simulink model "test_model"  (R2023a)
settings: Solver=ode5  StartTime=0.0  StopTime=10  FixedStep=0.002  RelTol=1e-3
undefined symbols (not defined in the file or in its folder): f
libraries: sldrtlib x3, instrumentlib x1
settings Model: Creator=DELL  LastModifiedBy=DELL
settings HardwareCC: ProdBitPerLong=64  ProdHWDeviceType=Intel->x86-64 (Linux 64)
settings ModelReferenceCC: EnableRefExpFcnMdlSchedulingChecks=on
settings RTWCC: Description=Simulink Desktop Real-Time  SystemTargetFile=sldrt.tlc  TemplateMakefile=sldrt.tmf  RTWCompilerOptimization=on
settings CodeAppCC: MaxIdLength=95
settings SimulinkDesktopRealTimeCC: TargetLibSuffix=_sldrt.a  TargetPreCompLibLocation=C:\Program Files\MATLAB\R2023a\toolbox\sldrt\lib\win64

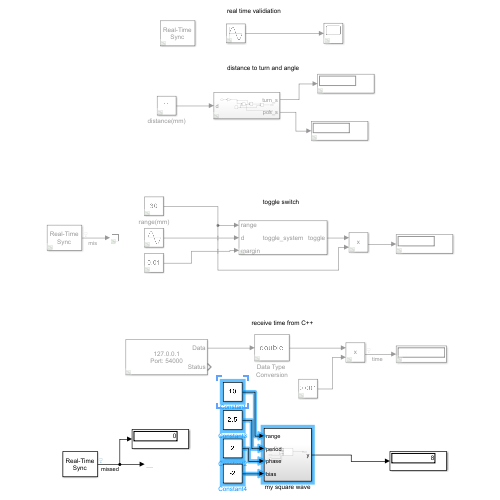
[thumbnail: Simulink's stored preview of the top-level diagram]
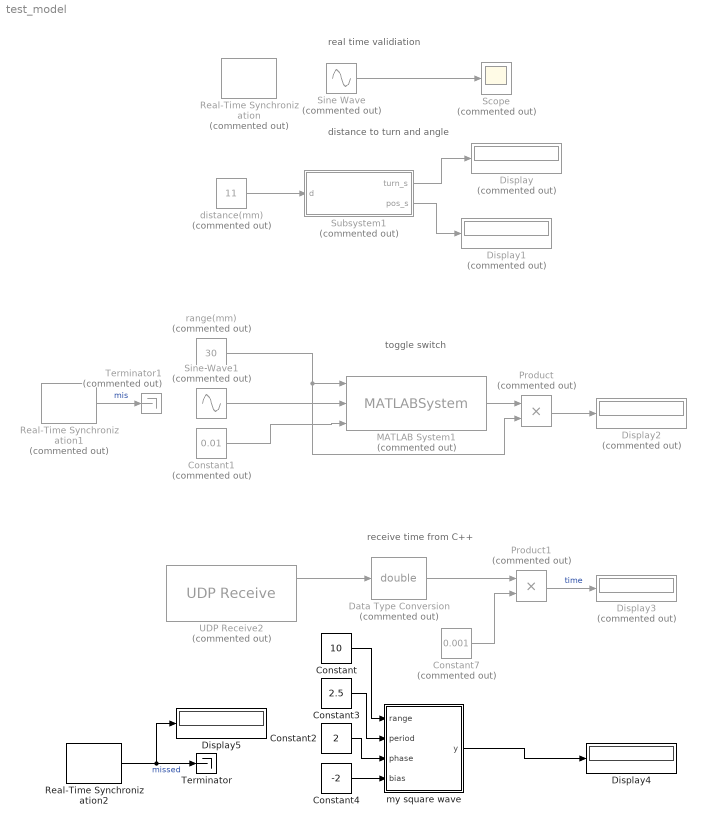
== system test_model ==
  note: real time validiation
  note: toggle switch
  note: distance to turn and angle
  note: receive time from C++
  Constant : Constant  Value=10
  Constant1 : Constant  Commented=on  Value=0.01
  Constant2 : Constant  Value=2
  Constant3 : Constant  Value=2.5
  Constant4 : Constant  Value=-2
  Constant7 : Constant  Commented=on  Value=0.001
  Data Type Conversion : DataTypeConversion  Commented=on  OutDataTypeStr=double  SaturateOnIntegerOverflow=off  RndMeth=Floor
  Display{,1..3} (4 alike) : Display  Commented=on
  Display4 : Display
  Display5 : Display
  MATLAB System1 : MATLABSystem  Commented=on  System=toggle_system  SimulateUsing=Code generation
      mask Type: toggle_system
      mask Display:
      | disp('toggle_system');
      | port_label('input',1,'range');
      | port_label('input',2,'d');
      | port_label('input',3,'margin');
      | port_label('output',1,'toggle');
  Product : Product  Commented=on
  Product1 : Product  Commented=on
  Real-Time Synchronization : sldrtlib/Real-Time Synchronization  Commented=on  SampleTime=0.01  MaxMissedTicks=10  ShowMissedTicks=off  YieldWhenWaiting=off
  Real-Time Synchronization1 : sldrtlib/Real-Time Synchronization  Commented=on  SampleTime=0.1  MaxMissedTicks=10  ShowMissedTicks=on  YieldWhenWaiting=off
  Real-Time Synchronization2 : sldrtlib/Real-Time Synchronization  SampleTime=0.002  MaxMissedTicks=inf  ShowMissedTicks=on  YieldWhenWaiting=off
  Scope : Scope  Commented=on
  Sine Wave : Sin  Commented=on
  Sine Wave1 : Sin  Commented=on  Amplitude=30  SampleTime=0
  Subsystem1 : Subsystem  Commented=on
  Terminator : Terminator
  Terminator1 : Terminator  Commented=on
  UDP Receive2 : instrumentlib/UDP Receive  Commented=on  LocalAddress=127.0.0.1  LocalPort=54000  EnablePortSharing=off  Host=127.0.0.1  Port=8080  GetLatestData=on  DataSize=1  DataType=uint32  ASCIIFormatting=%f,  Terminator=LF  CustomTerminator=10  ByteOrder=little-endian  EnableBlockingMode=off  Timeout=1  SampleTime=0.01  SimulateUsing=Interpreted execution
  distance(mm) : Constant  Commented=on  Value=11
  my square wave : Subsystem
  range(mm) : Constant  Commented=on  Value=30
  wires:
  Sine Wave/1 -> Scope/1
  distance(mm)/1 -> Subsystem1/1(d)
  Subsystem1/1(turn_s) -> Display/1
  Subsystem1/2(pos_s) -> Display1/1
  MATLAB System1/1 -> Product/1
  Sine Wave1/1 -> MATLAB System1/2
  Product1/1 -> Display3/1  "time"
  Data Type Conversion/1 -> Product1/1
  Constant7/1 -> Product1/2
  UDP Receive2/1 -> Data Type Conversion/1
  Product/1 -> Display2/1
  Constant1/1 -> MATLAB System1/3
  range(mm)/1 -> Product/2, MATLAB System1/1
  Real-Time Synchronization2/1 -> Display5/1, Terminator/1  "missed"
  Real-Time Synchronization1/1 -> Terminator1/1  "mis"
  Constant/1 -> my square wave/1(range)
  Constant3/1 -> my square wave/2(period)
  Constant2/1 -> my square wave/3(phase)
  my square wave/1(y) -> Display4/1
  Constant4/1 -> my square wave/4(bias)

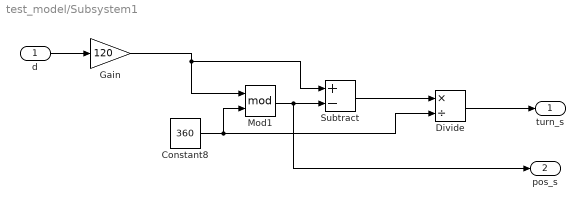
== system test_model/Subsystem1 ==
  d : Inport
  Constant8 : Constant  Value=360
  Divide : Product  Inputs=*/
  Gain : Gain  Gain=120
  Mod1 : Math  Operator=mod
  Subtract : Sum  Inputs=+-
  turn_s : Outport
  pos_s : Outport  Port=2
  wires:
  Constant8/1 -> Divide/2, Mod1/2
  Gain/1 -> Subtract/1, Mod1/1
  Mod1/1 -> pos_s/1, Subtract/2
  Subtract/1 -> Divide/1
  Divide/1 -> turn_s/1
  d/1 -> Gain/1

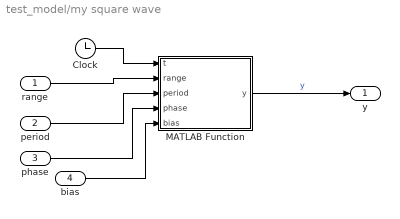
== system test_model/my square wave ==
  range : Inport
  period : Inport  Port=2
  phase : Inport  Port=3
  bias : Inport  Port=4
  Clock : Clock
  MATLAB Function : MATLAB Function  TreatAsAtomicUnit=on
  y : Outport
  wires:
  Clock/1 -> MATLAB Function/1(t)
  period/1 -> MATLAB Function/3(period)
  range/1 -> MATLAB Function/2(range)
  phase/1 -> MATLAB Function/4(phase)
  MATLAB Function/1(y) -> y/1  "y"
  bias/1 -> MATLAB Function/5(bias)

== matlab function test_model/my square wave/MATLAB Function ==
  data: t input; y output; range input; period input; phase input; bias input
function y = fcn(t,range,period,phase,bias)
t = t+phase;
remainder = mod(t,period);
t = t-remainder;
quotient = t/period;
if mod(quotient,2)==0
    y = range;
else
    y=-range;
end
y = y+bias;
